simulink model "LKAS_AutoSave_20200908_1055"  (R2018b)
settings: Solver=FixedStepDiscrete  StartTime=0.0  StopTime=10.0  FixedStep=0.01  RelTol=1e-3
InitFcn:
  | tmpVer = ver('MATLAB');
  | tmpVer = str2num(tmpVer.Version);
  | % -------------------------------------------------------------------
  | %  MATLAB file generated by Simulink.saveVars on 21-Nov-2019 10:06:14
  | %  MATLAB version: 7.13.0.564 (R2011b)
  | % -------------------------------------------------------------------
  | 
  | 
  | SInt16 = Simulink.AliasType;
  | SInt16.Description = 'Num';
  | if (tmpVer > 7.11)
  | 	SInt16.DataScope = 'Auto';
  | end
  | SInt16.HeaderFile = 'Rte_Type.h';
  | SInt16.BaseType = 'int16';
  | 
  | SInt32 = Simulink.AliasType;
  | SInt32.Description = 'Num';
  | if (tmpVer > 7.11)
  | 	SInt32.DataScope = 'Auto';
  | end
  | SInt32.HeaderFile = 'Rte_Type.h';
  | SInt32.BaseType = 'int32';
  | 
  | SInt8 = Simulink.AliasType;
  | SInt8.Description = 'Num';
  | if (tmpVer > 7.11)
  | 	SInt8.DataScope = 'Auto';
  | end
  | SInt8.HeaderFile = 'Rte_Type.h';
  | SInt8.BaseType = 'int8';
  | 
  | T_A_m2_1024_1_u32 = Simulink.NumericType;
  | T_A_m2_1024_1_u32.Description = 'm2 (square meters  (m2))';
  | if (tmpVer > 7.11)
  | 	T_A_m2_1024_1_u32.DataScope = 'Auto';
  | end
  | T_A_m2_1024_1_u32.HeaderFile = 'Rte_Type.h';
  | T_A_m2_1024_1_u32.DataTypeMode = 'Fixed-point: slope and bias scaling';
  | T_A_m2_1024_1_u32.SignednessBool = false;
  | T_A_m2_1024_1_u32.WordLength = 32;
  | T_A_m2_1024_1_u32.FixedExponent = -10;
  | T_A_m2_1024_1_u32.SlopeAdjustmentFactor = 1;
  | T_A_m2_1024_1_u32.Bias = 0;
  | T_A_m2_1024_1_u32.DataTypeOverride = 'Inherit';
  | T_A_m2_1024_1_u32.IsAlias = true;
  | 
  | T_A_m2_65536_1_u16 = Simulink.NumericType;
  | T_A_m2_65536_1_u16.Description = 'm2 (square meters  (m2))';
  | if (tmpVer > 7.11)
  | 	T_A_m2_65536_1_u16.DataScope = 'Auto';
  | end
  | T_A_m2_65536_1_u16.HeaderFile = 'Rte_Type.h';
  | T_A_m2_65536_1_u16.DataTypeMode = 'Fixed-point: slope and bias scaling';
  | T_A_m2_65536_1_u16.SignednessBool = false;
  | T_A_m2_65536_1_u16.WordLength = 16;
  | T_A_m2_65536_1_u16.FixedExponent = -16;
  | T_A_m2_65536_1_u16.SlopeAdjustmentFactor = 1;
  | T_A_m2_65536_1_u16.Bias = 0;
  | T_A_m2_65536_1_u16.DataTypeOverride = 'Inherit';
  | ... (+4598 lines)
StopFcn:
  | clear  T_A_m2_1024_1_u32 T_A_m2_65536_1_u16 T_A_m2_Float32 T_A_mm2_10_1_u16 T_A_mm2_4_1_s16 T_A_mm2_Float32 T_Cnt_Num_10_1_u32 T_Cnt_Num_1_1_s16 T_Cnt_Num_1_1_s32 T_Cnt_Num_1_1_s8 T_Cnt_Num_1_1_u16 T_Cnt_Num_1_1_u32 T_Cnt_Num_1_1_u8 T_E_J_1_1_s32 T_E_J_Float32 T_E_kJ_128_1_s32 T_E_kJ_Float32 T_E_kwh_10_1_u16 T_E_kwh_Float32 T_Epl_kwhpkm_100_1_u16 T_Epl_kwhpkm_Float32 T_F_N_1_1_s16 T_F_N_Float32 T_I_A_1000_1_u16 T_I_A_1048576_1_s32 T_I_A_2048_1_s16 T_I_A_32_1_s16 T_I_A_Float32 T_I_mA_1_1_s16 T_I_mA_32768_128_s16 T_I_mA_Float32 T_J_kgpm2_128_1_u16 T_J_kgpm2_Float32 T_K_NA_1000_1_s16 T_K_NA_100_1_s16 T_K_NA_100_1_u16 T_K_NA_1024_1_s16 T_K_NA_1024_1_u16 T_K_NA_128_1_s16 T_K_NA_128_1_u16 T_K_NA_128_1_u8 T_K_NA_16777216_1_u32 T_K_NA_16_1_s16 T_K_NA_16_1_u16 T_K_NA_16_1_u8 T_K_NA_1_16_u16 T_K_NA_1_1_s16 T_K_NA_1_1_u16 T_K_NA_1_1_u8 T_K_NA_32768_1_s16 T_K_NA_32768_1_u16 T_K_NA_32_1_s8 T_K_NA_4096_1_u16 T_K_NA_4194304_1_s32 T_K_NA_4194304_1_u16 T_K_NA_65536_1_s32 T_K_NA_65536_1_u16 T_K_NA_8192_1_s16 T_K_NA_8_1_s16 T_K_NA_Float32 T_M_Nm_16_1_s16 T_M_Nm_1_1_s16 T_M_Nm_32768_1_s16 T_M_Nm_32_1_s16 T_M_Nm_4_1_s16 T_M_Nm_512_1_s16 T_M_Nm_Float32 T_P_W_1_4_s16 T_P_W_1_8_s16 T_P_W_Float32 T_P_kW_128_1_s16 T_P_kW_1_8_s16 T_P_kW_8_1_s32 T_P_kW_Float32 T_Pct_pct_1024_1_s32 T_Pct_pct_1024_1_u32 T_Pct_pct_10_1_s16 T_Pct_pct_10_1_u32 T_Pct_pct_128_100_s8 T_Pct_pct_1_1_s16 T_Pct_pct_1_4_u8 T_Pct_pct_255_100_u16 T_Pct_pct_255_100_u8 T_Pct_pct_256_1_s16 T_Pct_pct_256_1_u16 T_Pct_pct_65535_100_u16 T_Pct_pct_Float32 T_R_ohm_1024_1_s16 T_R_ohm_32_1_s16 T_R_ohm_Float32 T_TK_K_16_1_s16 T_TK_K_Float32 T_T_degC_10_400_1_u16 T_T_degC_16_1_s16 T_T_degC_1_40_1_u8 T_T_degC_2_80_1_u8 T_T_degC_Float32 T_U_V_1000_1_u16 T_U_V_10_1_u8 T_U_V_200_1_u8 T_U_V_32_1_s16 T_U_V_4096_1_s16 T_U_V_512_1_s16 T_U_V_65535_8_u16 T_U_V_8192_1_u16 T_U_V_Float32 T_U_mV_1_1_s16 T_U_mV_256_20_u16 T_U_mV_Float32 T_V_l_256_1_s16 T_V_l_4096_1_s16 T_V_l_64_1_s16 T_V_l_65535_100_u16 T_V_l_Float32 T_V_ml_128_1_s16 T_V_ml_1_1_s16 T_V_ml_32768_1_s16 T_V_ml_Float32 T_V_ul_32_1_u16 T_V_ul_Float32 T_Vpl_clpkm_512_1_u16 T_Vpl_clpkm_Float32 T_a_kphps_16_1_s16 T_a_kphps_Float32 T_a_mps2_128_1_s16 T_a_mps2_Float32 T_c_MJpkg_256_1_s16 T_c_MJpkg_Float32 T_c_kJpgpK_1024_1_s16 T_c_kJpgpK_Float32 T_c_kJpkgpK_128_1_u16 T_c_kJpkgpK_Float32 T_chrg_Ah_1_1_s16 T_chrg_Ah_1_1_u16 T_chrg_Ah_1_1_u8 T_chrg_Ah_256_1_u16 T_chrg_Ah_4194304_1_s32 T_chrg_Ah_512_1_u16 T_chrg_Ah_8_1_u16 T_chrg_Ah_Float32 T_cmp_NA_100_1_s16 T_cmp_NA_128_1_s16 T_cmp_NA_16_1_s16 T_cmp_NA_32768_1_u16 T_cmp_NA_Float32 T_d2n_rpmps2_4_1_s16 T_d2n_rpmps2_Float32 T_dPct_pctps_16_1_s16 T_dPct_pctps_256_1_s16 T_dPct_pctps_Float32 T_dT_degCps_128_1_s16 T_dT_degCps_Float32 T_dV_lph_1_1_s16 T_dV_lph_Float32 T_dV_lpm_128_1_s16 T_dV_lpm_32_1_s16 T_dV_lpm_Float32 T_dV_lps_1024_1_u16 T_dV_lps_4_1_u16 T_dV_lps_Float32 T_dV_mlps_1024_1_s16 T_dV_mlps_Float32 T_d_BitField16 T_dm_gps_128_1_s16 T_dm_gps_128_1_u16 T_dm_gps_256_1_u16 T_dm_gps_Float32 T_dm_mgps_1_1_s16 T_dm_mgps_Float32 T_dn_rpmps_1_1_s16 T_dn_rpmps_2_1_s16 T_dn_rpmps_Float32 T_dp_Paps_1_1_s16 T_dp_Paps_Float32 T_dp_kPaps_1_1_s16 T_dp_kPaps_8_1_s16 T_dp_kPaps_Float32 T_dphi_degps_128_1_s16 T_dphi_degps_8_1_s16 T_dphi_degps_Float32 T_dr_ps_256_1_s16 T_dr_ps_Float32 T_drho_mgplps_1_2_s16 T_drho_mgplps_Float32 T_e_NA_1_1_u8 T_f_Hz_1_1_u16 T_f_Hz_1_1_u32 T_f_Hz_64_1_u16 T_f_Hz_8_1_s16 T_f_Hz_Float32 T_g_BitField32 T_l_km_16_1_s16 T_l_km_1_1_u16 T_l_km_1_1_u32 T_l_km_Float32 T_l_m_1024_1_s16 T_l_m_16_1_s16 T_l_m_1_1_u32 T_l_m_Float32 T_l_mm_16_1_s16 T_l_mm_1_1_u16 T_l_mm_4096_1_s16 T_l_mm_4_1_u8 T_l_mm_64_1_s16 T_l_mm_Float32 T_m_g_1_1_s16 T_m_g_2048_1_s16 T_m_g_32_1_u16 T_m_g_Float32 T_m_kg_1024_1_s16 T_m_kg_1_1_s16 T_m_kg_1_1_u32 T_m_kg_Float32 T_m_mg_128_1_s16 T_m_mg_32_1_s16 T_m_mg_Float32 T_n_rpm_1_1_s16 T_n_rpm_1_25_u8 T_n_rpm_256_50_u16 T_n_rpm_2_25_u8 T_n_rpm_4_1_u16 T_n_rpm_Float32 T_p_MPa_64_1_s16 T_p_MPa_Float32 T_p_Pa_1_1_s16 T_p_Pa_Float32 T_p_kPa_1_10_u16 T_p_kPa_1_1_s16 T_p_kPa_1_1_u8 T_p_kPa_256_1_u16 T_p_kPa_32_1_u16 T_p_kPa_64_1_s16 T_p_kPa_Float32 T_phi_deg_100_1_s16 T_phi_deg_1024_1_s16 T_phi_deg_128_1_s16 T_phi_deg_1_1_u8 T_phi_deg_256_1_s16 T_phi_deg_2_1_s8 T_phi_deg_32_1_s16 T_phi_deg_512_6_s32 T_phi_deg_Float32 T_phi_rad_2048_1_s16 T_phi_rad_Float32 T_r_NA_1024_1_s16 T_r_NA_1024_1_u16 T_r_NA_16384_1_s16 T_r_NA_16_1_s16 T_r_NA_256_1_s8 T_r_NA_256_1_u16 T_r_NA_32768_1_u16 T_r_NA_32_1_u16 T_r_NA_4096_1_s16 T_r_NA_65535_2_u16 T_r_NA_8192_1_u16 T_r_NA_Float32 T_rho_gpl_8192_1_s16 T_rho_gpl_Float32 T_rho_kgpm3_16_1_s16 T_rho_kgpm3_Float32 T_rho_mgpl_1_1_s16 T_rho_mgpl_64_1_s16 T_rho_mgpl_Float32 T_t_hour_1_1_s16 T_t_hour_Float32 T_t_m_1_1_u16 T_t_m_Float32 T_t_ms_1_1_s16 T_t_ms_1_1_u16 T_t_ms_1_1_u32 T_t_ms_4096_1_s16 T_t_ms_64_1_s16 T_t_ms_Float32 T_t_s_1000_1_s16 T_t_s_100_1_s16 T_t_s_10_1_s16 T_t_s_10_1_u16 T_t_s_1_1_s16 T_t_s_1_1_u16 T_t_s_1_1_u32 T_t_s_Float32 T_t_us_10_1_u32 T_t_us_1_1_s16 T_t_us_1_1_u32 T_t_us_1_4_u16 T_t_us_Float32 T_v_kph_1_1_u8 T_v_kph_64_1_s16 T_v_kph_64_1_u16 T_v_kph_Float32 T_v_mps_256_1_s16 T_v_mps_Float32 T_w_radps_32_1_s16 T_w_radps_Float32 T_y_BitField8 T_y_BitFieldDiagProgress T_y_BitFieldDiagStatus T_y_NA_1_1_u8 SInt16 SInt32 SInt8 T_BOOLEAN UInt16 UInt32 UInt8 s16 s32 s8 u16 u32 u8
model workspace (MAT data in the model file):
  MCOS : class17 (value not decoded)
  MCOS : class17 (value not decoded)
  MCOS : class17 (value not decoded)
  MCOS : class17 (value not decoded)
  MCOS : class17 (value not decoded)
  MCOS : class17 (value not decoded)
  MCOS : class17 (value not decoded)
  MCOS : class17 (value not decoded)
  MCOS : class17 (value not decoded)
  MCOS : class17 (value not decoded)
  MCOS : class17 (value not decoded)
  MCOS : class17 (value not decoded)
  MCOS : class17 (value not decoded)
  MCOS : class17 (value not decoded)
  MCOS : class17 (value not decoded)
  MCOS : class17 (value not decoded)
  MCOS : class17 (value not decoded)
  MCOS : class17 (value not decoded)
  MCOS : class17 (value not decoded)
  MCOS : class17 (value not decoded)
  MCOS : class17 (value not decoded)
  MCOS : class17 (value not decoded)
  MCOS : class17 (value not decoded)
  MCOS : class17 (value not decoded)
  MCOS : class17 (value not decoded)
  MCOS : class17 (value not decoded)
  MCOS : class17 (value not decoded)
  MCOS : class17 (value not decoded)
  MCOS : class17 (value not decoded)
  MCOS : class17 (value not decoded)
  MCOS : class17 (value not decoded)
  MCOS : class17 (value not decoded)
  MCOS : class17 (value not decoded)
  MCOS : class17 (value not decoded)
  MCOS : class17 (value not decoded)
  MCOS : class17 (value not decoded)
  MCOS : class17 (value not decoded)
  MCOS : class17 (value not decoded)
  MCOS : class17 (value not decoded)
  MCOS : class17 (value not decoded)
  MCOS : class17 (value not decoded)
  MCOS : class17 (value not decoded)
  MCOS : class17 (value not decoded)
  MCOS : class17 (value not decoded)
  MCOS : class17 (value not decoded)
  MCOS : class17 (value not decoded)
  MCOS : class17 (value not decoded)
  MCOS : class17 (value not decoded)
  MCOS : class17 (value not decoded)
  MCOS : class17 (value not decoded)
  MCOS : class17 (value not decoded)
  MCOS : class17 (value not decoded)
  MCOS : class17 (value not decoded)
  MCOS : class17 (value not decoded)
  MCOS : class17 (value not decoded)
  MCOS : class17 (value not decoded)
  MCOS : class17 (value not decoded)
  MCOS : class17 (value not decoded)
  MCOS : class17 (value not decoded)
  MCOS : class17 (value not decoded)
  MCOS : class17 (value not decoded)
  MCOS : class17 (value not decoded)
  MCOS : class17 (value not decoded)
  MCOS : class17 (value not decoded)
  MCOS : class17 (value not decoded)
  MCOS : class17 (value not decoded)
  MCOS : class17 (value not decoded)
  MCOS : class17 (value not decoded)
  MCOS : class17 (value not decoded)
  MCOS : class17 (value not decoded)
  MCOS : class17 (value not decoded)
  MCOS : class17 (value not decoded)
  MCOS : class17 (value not decoded)
  MCOS : class17 (value not decoded)
  MCOS : class17 (value not decoded)
  MCOS : class17 (value not decoded)
  MCOS : class17 (value not decoded)
  MCOS : class17 (value not decoded)
  MCOS : class17 (value not decoded)
  MCOS : class17 (value not decoded)
  MCOS : class17 (value not decoded)
  MCOS : class17 (value not decoded)
  MCOS : class17 (value not decoded)
  MCOS : class17 (value not decoded)
  MCOS : class17 (value not decoded)
  MCOS : class17 (value not decoded)
  MCOS : class17 (value not decoded)
  MCOS : class17 (value not decoded)
  MCOS : class17 (value not decoded)
undefined symbols (not defined in the file): LKA_CarWidth, LKA_SampleTime, LKA_StrRatio_C, LKA_Veh2CamL_C, LKA_Veh2CamW_C, LKA_WhlBaseL_C, LL_CompSWA_C, LL_CrvtPrvwT_C, LL_DesDvt_C, LL_DvtComp_C, LL_DvtPrvwT_C, LL_DvtSpdDet_vDvtSpdMin_C, LL_HdAgExT_C, LL_HdAgPrvwT_C, LL_LAccMax_C, LL_LAccRMax_C, LL_LDW_EarliestWarnLine_C, LL_LDW_LatestWarnLine_C, LL_LDWS_SUPPRESS_HEADING, LL_LFClb_TFC_DiffCtlBalance, LL_LFClb_TFC_DiffCtrlMaxSWA, LL_LFClb_TFC_DiffCtrlRatio, LL_LFClb_TFC_facmGainLutGain1_C, LL_LFClb_TFC_facmGainLutGain2_C, LL_LFClb_TFC_facmIntegRatio, LL_LFClb_TFC_facmKlat_C, LL_LFClb_TFC_FfCtlRatio_C, LL_LFClb_TFC_phiIntegCtlMaxSWA_C, LL_LFClb_TFC_tiKlatPrvwT_C, LL_LFClb_TFC_vGainLutVehSpdLwr_C, LL_LFClb_TFC_vGainLutVehSpdUpr_C, LL_LKA_EarliestWarnLine_C, LL_LKA_LatestWarnLine_C, LL_LKAExPrcs_ExitC0Dvt, LL_LKAExPrcs_ExitC0Swt, LL_LKAExPrcs_tiExitTime1, LL_LKAExPrcs_tiExitTime2, LL_LKAExPrcs_tiExitTime3, LL_LKAS_OUT_OF_CONTROL_LAT_VEL, LL_LKAS_OUT_OF_CONTROL_TTLC, LL_LKASWASyn_M0, LL_LKASWASyn_M1, LL_LKASWASyn_M2, LL_LKASWASyn_M3K, LL_LKASWASyn_SWAaddMax, LL_LKASWASyn_T2, LL_LKASWASyn_tiTrqSwaRtTime, LL_LKASWASyn_tiTrqSwaTime, LL_LKASWASyn_TrqMax, LL_LKASWASyn_TrqSwaAddSwt, LL_LKASWASyn_TrqSwaRateDiff, LL_LSpdCompT_C, LL_lStpLngth_C, LL_MAX_DELAY_EPSSTAR_TIME, LL_MAX_DRIVER_TORQUE_DISABLE, LL_MAX_DRIVER_TORQUE_ENABLE, LL_MAX_LANE_WIDTH_DISABLE, LL_MAX_LANE_WIDTH_ENABLE, LL_MAX_LAT_ACC_DISABLE, LL_MAX_LAT_ACC_ENABLE ... (+29)
libraries: simulink x134, dspstat3 x3, simulink_extras x1
(part 9 of 19)

== system LKAS_AutoSave_20200908_1055/LKAS/LL/LLOn/LKA/LKA Motion Planning (LKAMP) /Switching Condition (SwtCon) ==
  SwtCon_stLKAActvFlg : Inport
  SwtCon_bsLKAInPInfo : Inport  Port=2
  SwtCon_vVehSpd : Inport  Port=3
  SwtCon_lLaneWidth_C : Inport  Port=4
  SwtCon_lCarWidth_C : Inport  Port=5
  SwtCon_tiHdAgExTime_C : Inport  Port=6
  SwtCon_tiLSpdCompT_C : Inport  Port=7
  Bus Selector1 : BusSelector  OutputSignals=Pr_bsPrInfo.bsPrCrvtInfo.crPrvwCrvt
  Ending Heading Angle Determination (EndHdAgDet) : Subsystem
  If : If  IfExpression=u1==1  ElseIfExpressions=u1==2
  If Action Subsystem : Subsystem  TreatAsAtomicUnit=on
  If Action Subsystem1 : Subsystem  TreatAsAtomicUnit=on
  If Action Subsystem2 : Subsystem  TreatAsAtomicUnit=on
  Merge : Merge  Inputs=3
  Signal Latching : Subsystem  mask(Signal Latching:){LatchTime=1}
      mask prompts: LatchTime "Latch time(-):"
      mask help:
      | If the latch time is not reached, the input signal will just go through the block. If the latch time is reached, the output will be held and do not change again. The latch time is described with the number of the sampling time.
      | ----vcdc.ascl@jlu 19-01-15
  SwtCon_phiHdAgMax : Outport
  wires:
  Bus Selector1/1 -> Ending Heading Angle Determination (EndHdAgDet)/3(EndHdAgDet_crPrvwCrvt)  "<crPrvwCrvt>"
  SwtCon_bsLKAInPInfo/1 -> Bus Selector1/1
  SwtCon_tiLSpdCompT_C/1 -> Ending Heading Angle Determination (EndHdAgDet)/7(EndHdAgDet_tiLSpdCompT_C)
  Signal Latching/1(Out) -> SwtCon_phiHdAgMax/1
  SwtCon_stLKAActvFlg/1 -> Ending Heading Angle Determination (EndHdAgDet)/1(EndHdAgDet_stLKAActvFlg), If/1
  Merge/1 -> Signal Latching/1(In)
  Ending Heading Angle Determination (EndHdAgDet)/1(EndHdAgDet_phiHdAgMax) -> If Action Subsystem/1(In1), If Action Subsystem1/1(In1)
  SwtCon_vVehSpd/1 -> Ending Heading Angle Determination (EndHdAgDet)/2(EndHdAgDet_vVehSpd)
  SwtCon_tiHdAgExTime_C/1 -> Ending Heading Angle Determination (EndHdAgDet)/6(EndHdAgDet_tiHdAgExTime_C)
  SwtCon_lCarWidth_C/1 -> Ending Heading Angle Determination (EndHdAgDet)/5(EndHdAgDet_lCarWidth_C)
  SwtCon_lLaneWidth_C/1 -> Ending Heading Angle Determination (EndHdAgDet)/4(EndHdAgDet_lLaneWidth_C)
  If Action Subsystem2/1(Out1) -> Merge/3
  If/3 -> If Action Subsystem2/Action
  If Action Subsystem1/1(Out1) -> Merge/2
  If/2 -> If Action Subsystem1/Action
  If Action Subsystem/1(Out1) -> Merge/1
  If/1 -> If Action Subsystem/Action

== system LKAS_AutoSave_20200908_1055/LKAS/LL/LLOn/LKA/LKA SWA Limit (LKASWALim)/Rate Limiter Dynamic  ==
  note: Y(k)
  note: U(k)
  up : Inport
  u : Inport  Port=2
  lo : Inport  Port=3
  Add1 : Sum  OutDataTypeStr=uint16
  Constant : Constant  OutDataTypeStr=uint16  SampleTime=-1
  Delay Input2 : UnitDelay  Description=Store in Global RAM  DisableCoverage=on  SampleTime=-1
  Difference Inputs1 : Sum  Description=Add in CPU  DisableCoverage=on  Inputs=+-  OutDataTypeStr=Inherit: Inherit via back propagation
  Difference Inputs2 : Sum  Description=Add in CPU  OutDataTypeStr=Inherit: Inherit via back propagation
  LatchTime_SY : Constant  OutDataTypeStr=uint16  SampleTime=-1
  Memory : Memory  InheritSampleTime=on
  Relational Operator : RelationalOperator  Operator=<=  OutDataTypeStr=boolean  RndMeth=Nearest
  Saturation Dynamic : simulink/Discontinuities/Saturation Dynamic  OutMin=[]  OutMax=[]  OutDataTypeStr=Inherit: Same as second input  OutDataType=fixdt(1, 16)  OutScaling=2^-10  DoSatur=off
  Saturation2 : Saturate  UpperLimit=10000  LowerLimit=0  OutDataTypeStr=uint16
  Switch : Switch  Criteria=u2 > Threshold
  delta fall limit : Product  DisableCoverage=on  Inputs=**  OutDataTypeStr=Inherit: Inherit via back propagation  SaturateOnIntegerOverflow=on
  delta rise limit : Product  DisableCoverage=on  Inputs=**  OutDataTypeStr=Inherit: Inherit via back propagation  SaturateOnIntegerOverflow=on
  sample time : SampleTimeMath  DisableCoverage=on  TsampMathOp=Ts Only  weightValue=1
  Y : Outport
  wires:
  u/1 -> sample time/1, Switch/1, Difference Inputs1/1
  sample time/1 -> delta fall limit/2, delta rise limit/2
  lo/1 -> delta fall limit/1
  up/1 -> delta rise limit/1
  delta rise limit/1 -> Saturation Dynamic/1
  Difference Inputs2/1 -> Y/1, Delay Input2/1
  Saturation Dynamic/1 -> Difference Inputs2/1
  Switch/1 -> Difference Inputs2/2, Difference Inputs1/2  "Y(k-1)"
  Difference Inputs1/1 -> Saturation Dynamic/2  "( U(k) - Y(k-1) )"
  delta fall limit/1 -> Saturation Dynamic/3
  Add1/1 -> Relational Operator/1, Saturation2/1
  Memory/1 -> Add1/2
  Saturation2/1 -> Memory/1
  LatchTime_SY/1 -> Relational Operator/2
  Constant/1 -> Add1/1
  Relational Operator/1 -> Switch/2
  Delay Input2/1 -> Switch/3  "Y(k-1)"

== system LKAS_AutoSave_20200908_1055/LKAS/LL/LLOn/LKA/Lane Following (LF)/Preview Information Calculation (PIC) ==
  PIC_bsLKAInPInfo : Inport
  Add : Sum
  Add1 : Sum
  Add2 : Sum
  Bus Creator1 : BusCreator  Inputs=5
  Bus Selector1 : BusSelector  OutputSignals=Pr_bsPrInfo.bsPrDvtInfo.lPrvwDvtLft,Pr_bsPrInfo.bsPrDvtInfo.lPrvwDvtRgt,Pr_bsPrInfo.bsPrHdAgInfo.phiPrvwHdAgLft,Pr_bsPrInfo.bsPrHdAgInfo.phiPrvwHdAgRgt,Pr_bsPrInfo.bsPrCrvtInfo.crPrvwCrvtLft,Pr_bsPrInfo.bsPrCrvtInfo.crPrvwCrvtRgt,TTLC_bsTTLCInfo.vLft,TTLC_bsTTLCInfo.vRgt
  Gain : Gain  Gain=0.5
  Gain1 : Gain  Gain=0.5
  Gain2 : Gain  Gain=0.5
  PIC_bsPrvwInfo : Outport
  wires:
  Bus Creator1/1 -> PIC_bsPrvwInfo/1
  PIC_bsLKAInPInfo/1 -> Bus Selector1/1
  Bus Selector1/1 -> Add1/1  "<lPrvwDvtLft>"
  Bus Selector1/2 -> Add1/2  "<lPrvwDvtRgt>"
  Add2/1 -> Gain1/1
  Gain1/1 -> Bus Creator1/3  "PIC_crPrvwCrvt"
  Bus Selector1/4 -> Add/2  "<phiPrvwHdAgRgt>"
  Add1/1 -> Gain2/1
  Gain/1 -> Bus Creator1/2  "PIC_phiPrvwHdAg"
  Bus Selector1/6 -> Add2/2  "<crPrvwCrvtRgt>"
  Add/1 -> Gain/1
  Bus Selector1/3 -> Add/1  "<phiPrvwHdAgLft>"
  Bus Selector1/5 -> Add2/1  "<crPrvwCrvtLft>"
  Bus Selector1/7 -> Bus Creator1/4  "<vLft>"
  Bus Selector1/8 -> Bus Creator1/5  "<vRgt>"
  Gain2/1 -> Bus Creator1/1  "PIC_lPrvwDvt"

== system LKAS_AutoSave_20200908_1055/LKAS/LL/LLOn/LKA/Lane Following (LF)/Trajectory Following Control (TFC) ==
  TFC_bsPrvwInfo : Inport
  TFC_bsInInfoSyn : Inport  Port=2
  TFC_bsTFCClb : Inport  Port=3
  TFC_bsConstantClb : Inport  Port=4
  Bus Selector : BusSelector  OutputSignals=PIC_lPrvwDvt,PIC_phiPrvwHdAg,PIC_crPrvwCrvt
  Bus Selector1 : BusSelector  OutputSignals=LL_LFClb_TFC_tiKlatPrvwT_C,LL_LFClb_TFC_facmKlat_C,LL_LFClb_TFC_vGainLutVehSpdLwr_C,LL_LFClb_TFC_vGainLutVehSpdUpr_C,LL_LFClb_TFC_facmGainLutGain1_C,LL_LFClb_TFC_facmGainLutGain2_C,LL_LFClb_TFC_phiIntegCtlMaxSWA_C,LL_LFClb_TFC_facmIntegRatio,LL_LFClb_TFC_DiffCtrlRatio,LL_LFClb_TFC_DiffCtrlMaxSWA,LL_LFClb_TFC_DiffCtlBalance,LL_LFClb_TFC_FfCtlRatio_C
  Bus Selector2 : BusSelector  OutputSignals=LKA_WhlBaseL_C,LKA_StrRatio_C
  Bus Selector3 : BusSelector  OutputSignals=bsLaneInfo.bsL0Info,bsLaneInfo.bsR0Info,bsVehMovInfo.ESC_VehSpd
  Feedback Control (FbCtl) : Subsystem
  Feedforward Control (FfCtl) : Subsystem
  TFC_phiFfSWACmd : Outport
  TFC_phiPropSWACmd : Outport  Port=2
  TFC_phiIntegSWACmd : Outport  Port=3
  TFC_phiDiffSWACmd : Outport  Port=4
  wires:
  Feedback Control (FbCtl)/3(FbCtl_phiFbDiffCtlSWA) -> TFC_phiDiffSWACmd/1
  Bus Selector3/2 -> Feedback Control (FbCtl)/2(FbCtl_bsR0Info)  "<bsR0Info>"
  Bus Selector3/1 -> Feedback Control (FbCtl)/1(FbCtl_bsL0Info)  "<bsL0Info>"
  TFC_bsInInfoSyn/1 -> Bus Selector3/1
  Bus Selector/3 -> Feedforward Control (FfCtl)/3(FfCtl_crPrvwCrvt), Feedback Control (FbCtl)/6(FbCtl_crPrvwCrvt)  "<PIC_crPrvwCrvt>"
  Feedforward Control (FfCtl)/1(FfCtl_phiFfSWA) -> TFC_phiFfSWACmd/1  "phiFfSWA"
  Feedback Control (FbCtl)/1(FbCtl_phiFbPropCtlSWA) -> TFC_phiPropSWACmd/1
  TFC_bsPrvwInfo/1 -> Bus Selector/1  "bsPrvwInfo"
  Bus Selector/1 -> Feedback Control (FbCtl)/4(FbCtl_lPrvwDvt)  "<PIC_lPrvwDvt>"
  Bus Selector/2 -> Feedback Control (FbCtl)/5(FbCtl_phiPrvwHdAg)  "<PIC_phiPrvwHdAg>"
  TFC_bsTFCClb/1 -> Bus Selector1/1
  Bus Selector1/1 -> Feedback Control (FbCtl)/7(FbCtl_tiKlatPrvwT_C)  "<LL_LFClb_TFC_tiKlatPrvwT_C>"
  Bus Selector1/2 -> Feedback Control (FbCtl)/8(FbCtl_facmKlat_C)  "<LL_LFClb_TFC_facmKlat_C>"
  Bus Selector3/3 -> Feedback Control (FbCtl)/3(FbCtl_vVehSpd), Feedforward Control (FfCtl)/2(FfCtl_vVehSpd)  "<ESC_VehSpd>"
  Bus Selector1/3 -> Feedback Control (FbCtl)/9(FbCtl_vVehSpdLimLwr_C)  "<LL_LFClb_TFC_vGainLutVehSpdLwr_C>"
  Bus Selector1/4 -> Feedback Control (FbCtl)/10(FbCtl_vVehSpdLimUpr_C)  "<LL_LFClb_TFC_vGainLutVehSpdUpr_C>"
  Bus Selector1/5 -> Feedback Control (FbCtl)/11(FbCtl_facmGainLimLwr_C)  "<LL_LFClb_TFC_facmGainLutGain1_C>"
  Bus Selector1/6 -> Feedback Control (FbCtl)/12(FbCtl_facmGainLimUpr_C)  "<LL_LFClb_TFC_facmGainLutGain2_C>"
  Bus Selector2/1 -> Feedforward Control (FfCtl)/4(FfCtl_lWhlBase_SY)  "<LKA_WhlBaseL_C>"
  Bus Selector2/2 -> Feedforward Control (FfCtl)/5(FfCtl_rTraRatio_C)  "<LKA_StrRatio_C>"
  TFC_bsConstantClb/1 -> Bus Selector2/1
  Bus Selector1/12 -> Feedforward Control (FfCtl)/1(FfCtl_FfCtlRatio_C)  "<LL_LFClb_TFC_FfCtlRatio_C>"
  Bus Selector1/7 -> Feedback Control (FbCtl)/13(FbCtl_phiIntegCtlMaxSWA_C)  "<LL_LFClb_TFC_phiIntegCtlMaxSWA_C>"
  Bus Selector1/8 -> Feedback Control (FbCtl)/14(FbCtl_facmIntegRatio)  "<LL_LFClb_TFC_facmIntegRatio>"
  Feedback Control (FbCtl)/2(FbCtl_phiFbIntegCtlSWA) -> TFC_phiIntegSWACmd/1
  Bus Selector1/10 -> Feedback Control (FbCtl)/16(FbCtl_DiffCtlMaxSWA)  "<LL_LFClb_TFC_DiffCtrlMaxSWA>"
  Bus Selector1/9 -> Feedback Control (FbCtl)/15(FbCtl_DiffCtlRatioIn)  "<LL_LFClb_TFC_DiffCtrlRatio>"
  Bus Selector1/11 -> Feedback Control (FbCtl)/17(FbCtl_DiffCtlBalance)  "<LL_LFClb_TFC_DiffCtlBalance>"

== system LKAS_AutoSave_20200908_1055/LKAS/LL/LLOn/LKA/Plan To LaneFollowing (PTLF)/InsideJudge ==
  Flg : Inport
  Crvt : Inport  Port=2
  Compare To Constant : simulink/Logic and Bit Operations/Compare To Constant  relop===  const=1  OutDataTypeStr=boolean
  Compare To Constant1 : simulink/Logic and Bit Operations/Compare To Constant  relop===  const=2  OutDataTypeStr=boolean
  Constant : Constant  Value=0.001  OutDataTypeStr=single
  Constant3 : Constant  Value=-0.001  OutDataTypeStr=single
  Logical Operator : Logic  AllPortsSameDT=off  OutDataTypeStr=boolean
  Logical Operator1 : Logic  AllPortsSameDT=off  OutDataTypeStr=boolean
  Logical Operator2 : Logic  Operator=OR  AllPortsSameDT=off  OutDataTypeStr=boolean
  Relational Operator : RelationalOperator  OutDataTypeStr=boolean  RndMeth=Simplest
  Relational Operator1 : RelationalOperator  Operator=<=  OutDataTypeStr=boolean  RndMeth=Simplest
  Out1 : Outport
  wires:
  Compare To Constant/1 -> Logical Operator1/1  "LeftActive"
  Logical Operator1/1 -> Logical Operator2/1
  Logical Operator/1 -> Logical Operator2/2
  Flg/1 -> Compare To Constant1/1, Compare To Constant/1
  Relational Operator/1 -> Logical Operator/2  "RightCrvt"
  Compare To Constant1/1 -> Logical Operator/1  "RightActive"
  Constant/1 -> Relational Operator/2
  Relational Operator1/1 -> Logical Operator1/2  "LeftCrvt"
  Constant3/1 -> Relational Operator1/2
  Logical Operator2/1 -> Out1/1
  Crvt/1 -> Relational Operator1/1, Relational Operator/1

== system LKAS_AutoSave_20200908_1055/LKAS/LL/LLOn/LKA/Plan To LaneFollowing (PTLF)/InsideJudge1 ==
  Flg : Inport
  HdAgLft : Inport  Port=2
  HdAgRgt : Inport  Port=3
  T1 : Inport  Port=4
  Plan : Inport  Port=5
  Time : Inport  Port=6
  If : If  IfExpression=u1 == 1  ElseIfExpressions=u1 == 2
  If Action Subsystem : Subsystem  TreatAsAtomicUnit=on
  If Action Subsystem1 : Subsystem  TreatAsAtomicUnit=on
  If Action Subsystem2 : Subsystem  TreatAsAtomicUnit=on
  Merge : Merge  Inputs=3  InitialOutput=1
  Merge1 : Merge  Inputs=3  InitialOutput=0
  T1_1 : Outport
  Plan_1 : Outport  Port=2
  wires:
  Flg/1 -> If/1
  If/1 -> If Action Subsystem/Action
  If/2 -> If Action Subsystem1/Action
  If/3 -> If Action Subsystem2/Action
  HdAgLft/1 -> If Action Subsystem/3(HdAgLft)
  If Action Subsystem/1(T1_1) -> Merge/1
  If Action Subsystem1/1(T1_1) -> Merge/2
  If Action Subsystem2/1(T1_1) -> Merge/3
  If Action Subsystem/2(Plan_1) -> Merge1/1
  If Action Subsystem1/2(Plan_1) -> Merge1/2
  If Action Subsystem2/2(Plan_1) -> Merge1/3
  T1/1 -> If Action Subsystem/1(T1), If Action Subsystem1/1(T1), If Action Subsystem2/1(T1)
  Plan/1 -> If Action Subsystem/2(Plan), If Action Subsystem1/2(Plan), If Action Subsystem2/2(Plan)
  HdAgRgt/1 -> If Action Subsystem1/3(HdAgRgt)
  Merge/1 -> T1_1/1
  Merge1/1 -> Plan_1/1
  Time/1 -> If Action Subsystem1/4(Time), If Action Subsystem/4(Time)

== system LKAS_AutoSave_20200908_1055/LKAS/LL/LLOn/LKA/Plan To LaneFollowing (PTLF)/LowPass ==
  T : Inport
  u : Inport  Port=2
  dT : Inport  Port=3
  Add : Sum  Inputs=+-
  Add1 : Sum
  Add2 : Sum  OutDataTypeStr=single
  Divide : Product  Inputs=*/
  Divide1 : Product  Inputs=**
  Memory3 : Memory  InheritSampleTime=on
  SWACmdSyn_tiSmplT_C4 : Constant  OutDataTypeStr=single
  Saturation : Saturate  UpperLimit=50  LowerLimit=0
  Switch : Switch  Criteria=u2 > Threshold  Threshold=30
  Unit Delay : UnitDelay  SampleTime=-1
  y : Outport
  wires:
  Switch/1 -> Unit Delay/1, y/1
  Memory3/1 -> Add2/2
  Saturation/1 -> Memory3/1, Switch/2
  Add2/1 -> Saturation/1
  SWACmdSyn_tiSmplT_C4/1 -> Add2/1
  Add1/1 -> Switch/1
  Unit Delay/1 -> Add1/2, Add/2
  Divide1/1 -> Add1/1
  Add/1 -> Divide1/2
  Divide/1 -> Divide1/1
  u/1 -> Add/1, Switch/3
  dT/1 -> Divide/1
  T/1 -> Divide/2

== system LKAS_AutoSave_20200908_1055/LKAS/LL/LLOn/LKA/Plan To LaneFollowing (PTLF)/TickTime (TTime) ==
  Add2 : Sum  OutDataTypeStr=single
  Memory3 : Memory  InheritSampleTime=on
  Saturation : Saturate  UpperLimit=50  LowerLimit=0
  Out1 : Outport
  wires:
  Add2/1 -> Saturation/1
  Memory3/1 -> Add2/2
  Saturation/1 -> Out1/1, Memory3/1
  [LKA_SampleTime] -> Add2/1

== system LKAS_AutoSave_20200908_1055/LKAS/LL/LLOn/LKA/Plan To LaneFollowing (PTLF)/TimeGain ==
  Time : Inport
  T1 : Inport  Port=2
  TFC : Inport  Port=3
  Add1 : Sum
  Add2 : Sum  Inputs=+-
  Add3 : Sum  Inputs=-+
  Constant1 : Constant  Value=0  OutDataTypeStr=single
  Constant4 : Constant  OutDataTypeStr=single
  Divide : Product  Inputs=*/
  Divide8 : Product  Inputs=**
  Saturation4 : Saturate  UpperLimit=1  LowerLimit=0
  Out1 : Outport
  wires:
  Saturation4/1 -> Divide8/2
  Constant1/1 -> Add1/1, Add3/1
  Divide8/1 -> Add1/2
  Add1/1 -> Out1/1
  TFC/1 -> Divide/2
  T1/1 -> Add2/2
  Time/1 -> Add2/1
  Divide/1 -> Saturation4/1
  Add2/1 -> Divide/1
  Constant4/1 -> Add3/2
  Add3/1 -> Divide8/1

== system LKAS_AutoSave_20200908_1055/LKAS/LL/LLOn/LKA Input Processing (LKAInP)/Predicted Deviation Calculation (PrDvt)/Lane Information Selection (LaneInfoSel) ==
  LaneInfoSel_stLKAActvFlg : Inport
  LaneInfoSel_facmLftLane : Inport  Port=2
  LaneInfoSel_facmRgtLane : Inport  Port=3
  If : If  IfExpression=u1==1  ElseIfExpressions=u1==2
  If Action Subsystem1 : Subsystem  TreatAsAtomicUnit=on
  If Action Subsystem2 : Subsystem  TreatAsAtomicUnit=on
  If Action Subsystem3 : Subsystem  TreatAsAtomicUnit=on
  Merge : Merge  Inputs=3
  LaneInfoSel_facmActvLane : Outport
  wires:
  If/3 -> If Action Subsystem3/Action
  If Action Subsystem3/1(Out1) -> Merge/3
  If Action Subsystem1/1(Out1) -> Merge/2
  If/2 -> If Action Subsystem1/Action
  Merge/1 -> LaneInfoSel_facmActvLane/1
  If Action Subsystem2/1(Out1) -> Merge/1
  If/1 -> If Action Subsystem2/Action
  LaneInfoSel_stLKAActvFlg/1 -> If/1
  LaneInfoSel_facmLftLane/1 -> If Action Subsystem3/1(In1), If Action Subsystem2/1(In1)
  LaneInfoSel_facmRgtLane/1 -> If Action Subsystem3/2(In2), If Action Subsystem1/1(In1)

== system LKAS_AutoSave_20200908_1055/LKAS/LL/LLOn/LKA Input Processing (LKAInP)/Predicted Deviation Calculation (PrDvt)/Lane Information Selection (LaneInfoSel)1 ==
  LaneInfoSel_stLKAActvFlg : Inport
  LaneInfoSel_facmLftLane : Inport  Port=2
  LaneInfoSel_facmRgtLane : Inport  Port=3
  If : If  IfExpression=u1==1  ElseIfExpressions=u1==2
  If Action Subsystem1 : Subsystem  TreatAsAtomicUnit=on
  If Action Subsystem2 : Subsystem  TreatAsAtomicUnit=on
  If Action Subsystem3 : Subsystem  TreatAsAtomicUnit=on
  Merge : Merge  Inputs=3
  LaneInfoSel_facmActvLane : Outport
  wires:
  LaneInfoSel_facmRgtLane/1 -> If Action Subsystem1/1(In1), If Action Subsystem3/2(In2)
  LaneInfoSel_facmLftLane/1 -> If Action Subsystem2/1(In1), If Action Subsystem3/1(In1)
  LaneInfoSel_stLKAActvFlg/1 -> If/1
  If/1 -> If Action Subsystem2/Action
  If Action Subsystem2/1(Out1) -> Merge/1
  Merge/1 -> LaneInfoSel_facmActvLane/1
  If/2 -> If Action Subsystem1/Action
  If Action Subsystem1/1(Out1) -> Merge/2
  If Action Subsystem3/1(Out1) -> Merge/3
  If/3 -> If Action Subsystem3/Action

== system LKAS_AutoSave_20200908_1055/LKAS/LL/LLOn/LKA Input Processing (LKAInP)/Predicted Deviation Calculation (PrDvt)/Left Front Conner Deviation Calculation (LFCDvtCalc) ==
  PrdcDvt_bsPrHdAgInfo : Inport
  LFCDvtCalc_lDvt : Inport  Port=2
  LFCDvtCalc_lDvtComp_C : Inport  Port=3
  Add : Sum  Inputs=+-  OutDataTypeStr=single
  Add1 : Sum  OutDataTypeStr=single
  Add5 : Sum  OutDataTypeStr=single
  Bus Selector : BusSelector  OutputSignals=LKA_Veh2CamW_C,LKA_Veh2CamL_C
  Bus Selector2 : BusSelector  OutputSignals=phiHdAgLft
  Cos2 : Trigonometry  Operator=cos
  Divide : Product  Inputs=**
  Divide1 : Product  Inputs=**
  Gain1 : Gain  Gain=-1  OutDataTypeStr=single
  Sin : Trigonometry
  DvtCalc_lLftDvt : Outport
  wires:
  LFCDvtCalc_lDvt/1 -> Add/1
  LFCDvtCalc_lDvtComp_C/1 -> Add/2
  Add/1 -> Add1/1
  Bus Selector/1 -> Add1/2  "<LKA_Veh2CamW_C>"
  [LLClb_bsConstantClb] -> Bus Selector/1
  PrdcDvt_bsPrHdAgInfo/1 -> Bus Selector2/1
  Bus Selector/2 -> Divide1/1  "<LKA_Veh2CamL_C>"
  Bus Selector2/1 -> Sin/1, Cos2/1  "<phiHdAgLft>"
  Gain1/1 -> DvtCalc_lLftDvt/1
  Cos2/1 -> Divide/2
  Sin/1 -> Divide1/2
  Divide/1 -> Add5/1
  Divide1/1 -> Add5/2
  Add1/1 -> Divide/1
  Add5/1 -> Gain1/1

== system LKAS_AutoSave_20200908_1055/LKAS/LL/LLOn/LKA Input Processing (LKAInP)/Predicted Deviation Calculation (PrDvt)/Predicted Deviation Correction (PrdcDvtCor) ==
  PrdcDvtCor_bsPrdcHdAgInfo : Inport
  PrdcDvtCor_lPrvwDstZ : Inport  Port=2
  Bus Selector : BusSelector  OutputSignals=phiPrdcHdAgComp
  Divide2 : Product  Inputs=**  OutDataTypeStr=single
  PrdcDvtCor_lPrdcDvtCor : Outport
  wires:
  Bus Selector/1 -> Divide2/2  "<phiPrdcHdAgComp>"
  PrdcDvtCor_bsPrdcHdAgInfo/1 -> Bus Selector/1
  PrdcDvtCor_lPrvwDstZ/1 -> Divide2/1
  Divide2/1 -> PrdcDvtCor_lPrdcDvtCor/1

== system LKAS_AutoSave_20200908_1055/LKAS/LL/LLOn/LKA Input Processing (LKAInP)/Predicted Deviation Calculation (PrDvt)/Predicted Deviation of Left Lane Line (PrdcDvtLft) ==
  PrdcDvtLft_bsL0Info : Inport
  PrdcDvtLft_lPrvwDstZ : Inport  Port=2
  Add : Sum  Inputs=++++  AccumDataTypeStr=single
  Bus Selector : BusSelector  OutputSignals=L0_C0,L0_C1,L0_C2,L0_C3
  Product : Product  OutDataTypeStr=single  RndMeth=Zero
  Product3 : Product  OutDataTypeStr=single  RndMeth=Zero
  Product4 : Product  OutDataTypeStr=single  RndMeth=Zero
  Z*Z : Product  OutDataTypeStr=single  RndMeth=Zero
  Z*Z*Z : Product  OutDataTypeStr=single  RndMeth=Zero
  PrdcDvtLft_lPrdcDvtLft : Outport
  wires:
  Z*Z/1 -> Z*Z*Z/2, Product3/2
  Z*Z*Z/1 -> Product4/2
  Product4/1 -> Add/4
  Bus Selector/4 -> Product4/1  "<L0_C3>"
  Bus Selector/3 -> Product3/1  "<L0_C2>"
  Product3/1 -> Add/3
  Bus Selector/1 -> Add/1  "<L0_C0>"
  Product/1 -> Add/2
  Bus Selector/2 -> Product/1  "<L0_C1>"
  PrdcDvtLft_lPrvwDstZ/1 -> Z*Z/2, Product/2, Z*Z/1, Z*Z*Z/1
  PrdcDvtLft_bsL0Info/1 -> Bus Selector/1
  Add/1 -> PrdcDvtLft_lPrdcDvtLft/1

== system LKAS_AutoSave_20200908_1055/LKAS/LL/LLOn/LKA Input Processing (LKAInP)/Predicted Deviation Calculation (PrDvt)/Predicted Deviation of Left Line (PrdcDvtLft) ==
  PrdcDvtLft_bsPrdcHdAgInfo : Inport
  PrdcDvtLft_lPrdcDvtCor : Inport  Port=2
  PrdcDvtLft_lPrdcDvtLft : Inport  Port=3
  PrdcDvtLft_lDvtComp_C : Inport  Port=4
  " " : MATLAB Function  TreatAsAtomicUnit=on
  Add : Sum  Inputs=+-  AccumDataTypeStr=single  OutDataTypeStr=single
  Add1 : Sum  AccumDataTypeStr=single  OutDataTypeStr=single
  Add3 : Sum  AccumDataTypeStr=single  OutDataTypeStr=single
  Bus Selector : BusSelector  OutputSignals=phiPrvwTTLCHdAgLft,phiPrdcTTLCHdAg
  Bus Selector1 : BusSelector  OutputSignals=LKA_Veh2CamW_C,LKA_Veh2CamL_C
  Fcn3 : Fcn  Commented=on  Expr=u(2)*cos(u(1))+u(3)*sin(u(1))
  MATLAB Function : MATLAB Function  TreatAsAtomicUnit=on
  PrdcDvtLft_lDvtLft : Outport
  wires:
  Bus Selector1/1 -> " "/2(u2)  "<LKA_Veh2CamW_C>"
  Bus Selector/2 -> " "/1(u1)  "<phiPrdcTTLCHdAg>"
  Bus Selector/1 -> MATLAB Function/2(u2)  "<phiPrvwTTLCHdAgLft>"
  PrdcDvtLft_bsPrdcHdAgInfo/1 -> Bus Selector/1
  Add3/1 -> PrdcDvtLft_lDvtLft/1
  Add1/1 -> Add3/1  "PrvwDvtLft"
  Bus Selector1/2 -> " "/3(u3)  "<LKA_Veh2CamL_C>"
  PrdcDvtLft_lPrdcDvtCor/1 -> Add3/2  "PrdcDvtLft"
  MATLAB Function/1(y) -> Add1/1
  Add/1 -> MATLAB Function/1(u1)
  PrdcDvtLft_lDvtComp_C/1 -> Add/2
  PrdcDvtLft_lPrdcDvtLft/1 -> Add/1
  " "/1(y) -> Add1/2
  [LLClb_bsConstantClb] -> Bus Selector1/1

== system LKAS_AutoSave_20200908_1055/LKAS/LL/LLOn/LKA Input Processing (LKAInP)/Predicted Deviation Calculation (PrDvt)/Predicted Deviation of Right  Line (PrdcDvtRgt) ==
  PrdcDvtLft_bsPrdcHdAgInfo : Inport
  PrdcDvtLft_lPrdcDvtCor : Inport  Port=2
  PrdcDvtLft_lPrdcDvtLft : Inport  Port=3
  PrdcDvtLft_lDvtComp_C : Inport  Port=4
  " " : MATLAB Function  TreatAsAtomicUnit=on
  Add : Sum  Inputs=+-  AccumDataTypeStr=single  OutDataTypeStr=single
  Add2 : Sum  AccumDataTypeStr=single  OutDataTypeStr=single
  Add4 : Sum  Inputs=+-  AccumDataTypeStr=single  OutDataTypeStr=single
  Bus Selector : BusSelector  OutputSignals=phiPrvwTTLCHdAgRgt,phiPrdcTTLCHdAg
  Bus Selector1 : BusSelector  OutputSignals=LKA_Veh2CamW_C,LKA_Veh2CamL_C
  Fcn3 : Fcn  Commented=on  Expr=u(2)*cos(u(1))-u(3)*sin(u(1))
  MATLAB Function : MATLAB Function  TreatAsAtomicUnit=on
  PrdcDvtLft_lDvtRgt : Outport
  wires:
  Bus Selector/2 -> " "/1(u1)  "<phiPrdcTTLCHdAg>"
  Bus Selector/1 -> MATLAB Function/2(u2)  "<phiPrvwTTLCHdAgRgt>"
  PrdcDvtLft_bsPrdcHdAgInfo/1 -> Bus Selector/1
  Add2/1 -> PrdcDvtLft_lDvtRgt/1
  Bus Selector1/2 -> " "/3(u3)  "<LKA_Veh2CamL_C>"
  Bus Selector1/1 -> " "/2(u2)  "<LKA_Veh2CamW_C>"
  MATLAB Function/1(y) -> Add4/1
  Add/1 -> MATLAB Function/1(u1)
  PrdcDvtLft_lDvtComp_C/1 -> Add/2
  PrdcDvtLft_lPrdcDvtLft/1 -> Add/1
  Add4/1 -> Add2/1  "PrvwDvtRgt"
  " "/1(y) -> Add4/2
  PrdcDvtLft_lPrdcDvtCor/1 -> Add2/2  "PrdcDvtRgt"
  [LLClb_bsConstantClb] -> Bus Selector1/1

== system LKAS_AutoSave_20200908_1055/LKAS/LL/LLOn/LKA Input Processing (LKAInP)/Predicted Deviation Calculation (PrDvt)/Predicted Deviation of Right Lane Line (PrdcDvtRgt) ==
  PrdcDvtRgt_lPrvwDstZ : Inport
  PrdcDvtRgt_bsR0Info : Inport  Port=2
  Add : Sum  Inputs=++++  AccumDataTypeStr=single
  Bus Selector : BusSelector  OutputSignals=R0_C0,R0_C1,R0_C2,R0_C3
  Product : Product  OutDataTypeStr=single  RndMeth=Zero
  Product3 : Product  OutDataTypeStr=single  RndMeth=Zero
  Product4 : Product  OutDataTypeStr=single  RndMeth=Zero
  Z*Z : Product  OutDataTypeStr=single  RndMeth=Zero
  Z*Z*Z : Product  OutDataTypeStr=single  RndMeth=Zero
  PrdcDvtRgt_lPrdcDvtRgt : Outport
  wires:
  Z*Z/1 -> Z*Z*Z/2, Product3/2
  Z*Z*Z/1 -> Product4/2
  Product4/1 -> Add/4
  Bus Selector/4 -> Product4/1  "<R0_C3>"
  Bus Selector/3 -> Product3/1  "<R0_C2>"
  Product3/1 -> Add/3
  Bus Selector/1 -> Add/1  "<R0_C0>"
  Add/1 -> PrdcDvtRgt_lPrdcDvtRgt/1
  Product/1 -> Add/2
  Bus Selector/2 -> Product/1  "<R0_C1>"
  PrdcDvtRgt_lPrvwDstZ/1 -> Z*Z/2, Product/2, Z*Z/1, Z*Z*Z/1
  PrdcDvtRgt_bsR0Info/1 -> Bus Selector/1

== system LKAS_AutoSave_20200908_1055/LKAS/LL/LLOn/LKA Input Processing (LKAInP)/Predicted Deviation Calculation (PrDvt)/Right Front Conner Deviation Calculation (RFCDvtCalc) ==
  RFCDvtCalc_lDvtComp_C : Inport
  RFCDvtCalc_lDvt : Inport  Port=2
  PrdcDvt_bsPrHdAgInfo : Inport  Port=3
  Add : Sum  Inputs=+-  OutDataTypeStr=single
  Add1 : Sum  Inputs=+-  OutDataTypeStr=single
  Add5 : Sum  OutDataTypeStr=single
  Bus Selector1 : BusSelector  OutputSignals=LKA_Veh2CamW_C,LKA_Veh2CamL_C
  Bus Selector2 : BusSelector  OutputSignals=phiHdAgRgt
  Cos2 : Trigonometry  Operator=cos
  Divide : Product  Inputs=**
  Divide1 : Product  Inputs=**
  Sin : Trigonometry
  DvtCalc_lRgtDvt : Outport
  wires:
  RFCDvtCalc_lDvt/1 -> Add/1
  RFCDvtCalc_lDvtComp_C/1 -> Add/2
  Add/1 -> Add1/1
  PrdcDvt_bsPrHdAgInfo/1 -> Bus Selector2/1
  Bus Selector1/1 -> Add1/2  "<LKA_Veh2CamW_C>"
  Bus Selector1/2 -> Divide1/1  "<LKA_Veh2CamL_C>"
  [LLClb_bsConstantClb] -> Bus Selector1/1
  Add5/1 -> DvtCalc_lRgtDvt/1
  Sin/1 -> Divide1/2
  Divide1/1 -> Add5/2
  Bus Selector2/1 -> Cos2/1, Sin/1  "<phiHdAgRgt>"
  Cos2/1 -> Divide/2
  Add1/1 -> Divide/1
  Divide/1 -> Add5/1

== system LKAS_AutoSave_20200908_1055/LKAS/LL/LLOn/LKA Input Processing (LKAInP)/Predicted Deviation Calculation (PrDvt)/Z Calculation (ZCalc) ==
  ZCalc_vVehSpd : Inport
  ZCalc_tiDvtPrvwT_C : Inport  Port=2
  Divide : Product  Inputs=**  OutDataTypeStr=single
  kph to mps : Gain  Gain=1/3.6  OutDataTypeStr=single
  ZCalc_lPrvwDstZ : Outport
  wires:
  ZCalc_tiDvtPrvwT_C/1 -> Divide/2
  Divide/1 -> ZCalc_lPrvwDstZ/1
  kph to mps/1 -> Divide/1
  ZCalc_vVehSpd/1 -> kph to mps/1

== system LKAS_AutoSave_20200908_1055/LKAS/LL/LLOn/LKA Input Processing (LKAInP)/Predicted Heading Angle Calculation (PrHdAg)/Heading Angle (HdAg) ==
  HdAg_bsLaneInfo : Inport
  Add : Sum  AccumDataTypeStr=single
  Bus Selector : BusSelector  OutputSignals=bsLaneInfo.bsL0Info.L0_C1,bsLaneInfo.bsR0Info.R0_C1
  Gain : Gain  Gain=0.5
  HdAg_phiHdAg : Outport
  HdAg_phiHdAgLft : Outport  Port=2
  HdAg_phiHdAgRgt : Outport  Port=3
  wires:
  Add/1 -> Gain/1
  HdAg_bsLaneInfo/1 -> Bus Selector/1
  Bus Selector/1 -> HdAg_phiHdAgLft/1, Add/1  "<L0_C1>"
  Bus Selector/2 -> HdAg_phiHdAgRgt/1, Add/2  "<R0_C1>"
  Gain/1 -> HdAg_phiHdAg/1

== system LKAS_AutoSave_20200908_1055/LKAS/LL/LLOn/LKA Input Processing (LKAInP)/Predicted Heading Angle Calculation (PrHdAg)/Lane Information Selection (LaneInfoSel) ==
  LaneInfoSel_stLKAActvFlg : Inport
  LaneInfoSel_facmLftLane : Inport  Port=2
  LaneInfoSel_facmRgtLane : Inport  Port=3
  If : If  IfExpression=u1==1  ElseIfExpressions=u1==2
  If Action Subsystem1 : Subsystem  TreatAsAtomicUnit=on
  If Action Subsystem2 : Subsystem  TreatAsAtomicUnit=on
  If Action Subsystem3 : Subsystem  TreatAsAtomicUnit=on
  Merge : Merge  Inputs=3
  LaneInfoSel_facmActvLane : Outport
  wires:
  If/3 -> If Action Subsystem3/Action
  If Action Subsystem3/1(Out1) -> Merge/3
  If Action Subsystem1/1(Out1) -> Merge/2
  If/2 -> If Action Subsystem1/Action
  Merge/1 -> LaneInfoSel_facmActvLane/1
  If Action Subsystem2/1(Out1) -> Merge/1
  If/1 -> If Action Subsystem2/Action
  LaneInfoSel_stLKAActvFlg/1 -> If/1
  LaneInfoSel_facmLftLane/1 -> If Action Subsystem3/1(In1), If Action Subsystem2/1(In1)
  LaneInfoSel_facmRgtLane/1 -> If Action Subsystem3/2(In2), If Action Subsystem1/1(In1)

== system LKAS_AutoSave_20200908_1055/LKAS/LL/LLOn/LKA Input Processing (LKAInP)/Predicted Heading Angle Calculation (PrHdAg)/Lane Information Selection (LaneInfoSel)1 ==
  LaneInfoSel_stLKAActvFlg : Inport
  LaneInfoSel_facmLftLane : Inport  Port=2
  LaneInfoSel_facmRgtLane : Inport  Port=3
  If : If  IfExpression=u1==1  ElseIfExpressions=u1==2
  If Action Subsystem1 : Subsystem  TreatAsAtomicUnit=on
  If Action Subsystem2 : Subsystem  TreatAsAtomicUnit=on
  If Action Subsystem3 : Subsystem  TreatAsAtomicUnit=on
  Merge : Merge  Inputs=3
  LaneInfoSel_facmActvLane : Outport
  wires:
  LaneInfoSel_facmRgtLane/1 -> If Action Subsystem1/1(In1), If Action Subsystem3/2(In2)
  LaneInfoSel_facmLftLane/1 -> If Action Subsystem2/1(In1), If Action Subsystem3/1(In1)
  LaneInfoSel_stLKAActvFlg/1 -> If/1
  If/1 -> If Action Subsystem2/Action
  If Action Subsystem2/1(Out1) -> Merge/1
  Merge/1 -> LaneInfoSel_facmActvLane/1
  If/2 -> If Action Subsystem1/Action
  If Action Subsystem1/1(Out1) -> Merge/2
  If Action Subsystem3/1(Out1) -> Merge/3
  If/3 -> If Action Subsystem3/Action

== system LKAS_AutoSave_20200908_1055/LKAS/LL/LLOn/LKA Input Processing (LKAInP)/Predicted Heading Angle Calculation (PrHdAg)/Perdicted Heading Angle Compensation (PrdcHdAgComp) ==
  PrdcHdAgComp_vVehSpd : Inport
  PrdcHdAgComp_phiSWA : Inport  Port=2
  PrdcHdAgComp_tiHdAgPrvwT_C : Inport  Port=3
  Bus Selector : BusSelector  OutputSignals=LKA_StrRatio_C
  Divide1 : Product  Inputs=***  OutDataTypeStr=single
  Divide2 : Product  Inputs=*/  OutDataTypeStr=single
  Yaw Rate Stable Gain (YRSG) : Subsystem
  kph To mps : Gain  Gain=pi/180  OutDataTypeStr=single
  PrdcHdAgComp_phiPrdcHdAgComp : Outport
  wires:
  PrdcHdAgComp_vVehSpd/1 -> Yaw Rate Stable Gain (YRSG)/1(YRSG_vVehSpd)
  Yaw Rate Stable Gain (YRSG)/1(YRSG_dphiYRSG) -> Divide1/1
  kph To mps/1 -> Divide1/2
  PrdcHdAgComp_tiHdAgPrvwT_C/1 -> Divide1/3
  Divide1/1 -> Divide2/1
  Divide2/1 -> PrdcHdAgComp_phiPrdcHdAgComp/1
  PrdcHdAgComp_phiSWA/1 -> kph To mps/1
  Bus Selector/1 -> Divide2/2  "<LKA_StrRatio_C>"
  [LLClb_bsConstantClb] -> Bus Selector/1

== system LKAS_AutoSave_20200908_1055/LKAS/LL/LLOn/LKA Input Processing (LKAInP)/Predicted Heading Angle Calculation (PrHdAg)/Perdicted Heading Angle from Right Lane Line (PrdcHdAgRgt) ==
  PrdcHdAgRgt_lPrvwDstZ : Inport
  PrdcHdAgRgt_bsR0Info : Inport  Port=2
  Add : Sum  Inputs=+++  AccumDataTypeStr=single
  Bus Selector : BusSelector  OutputSignals=R0_C1,R0_C2,R0_C3
  Gain : Gain  Gain=2  OutDataTypeStr=single
  Gain1 : Gain  Gain=3  OutDataTypeStr=single
  Product3 : Product  OutDataTypeStr=single  RndMeth=Zero
  Product4 : Product  OutDataTypeStr=single  RndMeth=Zero
  Z*Z : Product  OutDataTypeStr=single  RndMeth=Zero
  PrdcHdAgRgt_phiPrdcHdAgRgt : Outport
  wires:
  Gain1/1 -> Product4/1
  Gain/1 -> Product3/1
  Z*Z/1 -> Product4/2
  Product4/1 -> Add/3
  Bus Selector/3 -> Gain1/1  "<R0_C3>"
  Bus Selector/2 -> Gain/1  "<R0_C2>"
  Product3/1 -> Add/2
  Bus Selector/1 -> Add/1  "<R0_C1>"
  PrdcHdAgRgt_lPrvwDstZ/1 -> Z*Z/2, Product3/2, Z*Z/1
  PrdcHdAgRgt_bsR0Info/1 -> Bus Selector/1
  Add/1 -> PrdcHdAgRgt_phiPrdcHdAgRgt/1

== system LKAS_AutoSave_20200908_1055/LKAS/LL/LLOn/LKA Input Processing (LKAInP)/Predicted Heading Angle Calculation (PrHdAg)/Perdicted Heading Angle from Right Lane Line (PrdcHdAgRgt)1 ==
  PrdcHdAgRgt_lPrvwDstZ : Inport
  PrdcHdAgRgt_bsR0Info : Inport  Port=2
  Add : Sum  Inputs=+++  AccumDataTypeStr=single
  Bus Selector : BusSelector  OutputSignals=R0_C1,R0_C2,R0_C3
  Gain : Gain  Gain=2  OutDataTypeStr=single
  Gain1 : Gain  Gain=3  OutDataTypeStr=single
  Product3 : Product  OutDataTypeStr=single  RndMeth=Zero
  Product4 : Product  OutDataTypeStr=single  RndMeth=Zero
  Z*Z : Product  OutDataTypeStr=single  RndMeth=Zero
  PrdcHdAgRgt_phiPrdcHdAgRgt : Outport
  wires:
  Add/1 -> PrdcHdAgRgt_phiPrdcHdAgRgt/1
  PrdcHdAgRgt_bsR0Info/1 -> Bus Selector/1
  PrdcHdAgRgt_lPrvwDstZ/1 -> Z*Z/1, Product3/2, Z*Z/2
  Bus Selector/1 -> Add/1  "<R0_C1>"
  Product3/1 -> Add/2
  Bus Selector/2 -> Gain/1  "<R0_C2>"
  Bus Selector/3 -> Gain1/1  "<R0_C3>"
  Product4/1 -> Add/3
  Z*Z/1 -> Product4/2
  Gain/1 -> Product3/1
  Gain1/1 -> Product4/1

== system LKAS_AutoSave_20200908_1055/LKAS/LL/LLOn/LKA Input Processing (LKAInP)/Predicted Heading Angle Calculation (PrHdAg)/Predicted Heading Angle from Left Lane Line (PrdcHdAgtLft) ==
  PrdcHdAgtLft_bsL0Info : Inport
  PrdcHdAgtLft_lPrvwDstZ : Inport  Port=2
  Add : Sum  Inputs=+++  AccumDataTypeStr=single
  Bus Selector : BusSelector  OutputSignals=L0_C1,L0_C2,L0_C3
  Gain : Gain  Gain=2  OutDataTypeStr=single
  Gain1 : Gain  Gain=3  OutDataTypeStr=single
  Product3 : Product  OutDataTypeStr=single  RndMeth=Zero
  Product4 : Product  OutDataTypeStr=single  RndMeth=Zero
  Z*Z : Product  OutDataTypeStr=single  RndMeth=Zero
  PrdcHdAgtLft_phiPrdcHdAgLft : Outport
  wires:
  Gain1/1 -> Product4/1
  Gain/1 -> Product3/1
  Z*Z/1 -> Product4/2
  Product4/1 -> Add/3
  Bus Selector/3 -> Gain1/1  "<L0_C3>"
  Bus Selector/2 -> Gain/1  "<L0_C2>"
  Product3/1 -> Add/2
  Bus Selector/1 -> Add/1  "<L0_C1>"
  PrdcHdAgtLft_lPrvwDstZ/1 -> Z*Z/2, Product3/2, Z*Z/1
  PrdcHdAgtLft_bsL0Info/1 -> Bus Selector/1
  Add/1 -> PrdcHdAgtLft_phiPrdcHdAgLft/1

== system LKAS_AutoSave_20200908_1055/LKAS/LL/LLOn/LKA Input Processing (LKAInP)/Predicted Heading Angle Calculation (PrHdAg)/Predicted Heading Angle from Left Lane Line (PrdcHdAgtLft)1 ==
  PrdcHdAgtLft_bsL0Info : Inport
  PrdcHdAgtLft_lPrvwDstZ : Inport  Port=2
  Add : Sum  Inputs=+++  AccumDataTypeStr=single
  Bus Selector : BusSelector  OutputSignals=L0_C1,L0_C2,L0_C3
  Gain : Gain  Gain=2  OutDataTypeStr=single
  Gain1 : Gain  Gain=3  OutDataTypeStr=single
  Product3 : Product  OutDataTypeStr=single  RndMeth=Zero
  Product4 : Product  OutDataTypeStr=single  RndMeth=Zero
  Z*Z : Product  OutDataTypeStr=single  RndMeth=Zero
  PrdcHdAgtLft_phiPrdcHdAgLft : Outport
  wires:
  Add/1 -> PrdcHdAgtLft_phiPrdcHdAgLft/1
  PrdcHdAgtLft_bsL0Info/1 -> Bus Selector/1
  PrdcHdAgtLft_lPrvwDstZ/1 -> Z*Z/1, Product3/2, Z*Z/2
  Bus Selector/1 -> Add/1  "<L0_C1>"
  Product3/1 -> Add/2
  Bus Selector/2 -> Gain/1  "<L0_C2>"
  Bus Selector/3 -> Gain1/1  "<L0_C3>"
  Product4/1 -> Add/3
  Z*Z/1 -> Product4/2
  Gain/1 -> Product3/1
  Gain1/1 -> Product4/1

== system LKAS_AutoSave_20200908_1055/LKAS/LL/LLOn/LKA Input Processing (LKAInP)/Predicted Heading Angle Calculation (PrHdAg)/Z Calculation (ZCalc) ==
  ZCalc_vVehSpd : Inport
  ZCalc_tiHdAgPrvwT_C : Inport  Port=2
  Divide : Product  Inputs=**  OutDataTypeStr=single
  kph to mps : Gain  Gain=1/3.6  OutDataTypeStr=single
  ZCalc_lPrvwDstZ : Outport
  wires:
  kph to mps/1 -> Divide/1
  Divide/1 -> ZCalc_lPrvwDstZ/1
  ZCalc_tiHdAgPrvwT_C/1 -> Divide/2
  ZCalc_vVehSpd/1 -> kph to mps/1

== system LKAS_AutoSave_20200908_1055/LKAS/LL/LLOn/LKA Input Processing (LKAInP)/Predicted Heading Angle Calculation (PrHdAg)/Z Calculation (ZCalc)1 ==
  ZCalc_vVehSpd : Inport
  ZCalc_tiHdAgPrvwT_C : Inport  Port=2
  Divide : Product  Inputs=**  OutDataTypeStr=single
  kph to mps : Gain  Gain=1/3.6  OutDataTypeStr=single
  ZCalc_lPrvwDstZ : Outport
  wires:
  ZCalc_vVehSpd/1 -> kph to mps/1
  ZCalc_tiHdAgPrvwT_C/1 -> Divide/2
  Divide/1 -> ZCalc_lPrvwDstZ/1
  kph to mps/1 -> Divide/1

== system LKAS_AutoSave_20200908_1055/LKAS/LL/LLOn/LKA Input Processing (LKAInP)/Previewed Curvature (PrCrvt)/Curvature Ahead of Left Lane Line (CrvtAhdLft) ==
  CrvtAhdLft_bsL0Info : Inport
  CrvtAhdLft_lPrvwDstZ : Inport  Port=2
  Add : Sum  AccumDataTypeStr=single
  Bus Selector : BusSelector  OutputSignals=L0_C2,L0_C3
  Gain : Gain  Gain=2  OutDataTypeStr=single
  Gain1 : Gain  Gain=6  OutDataTypeStr=single
  Product : Product  OutDataTypeStr=single  RndMeth=Zero
  CrvtAhdLft_crCrvtAhdLft : Outport
  wires:
  Add/1 -> CrvtAhdLft_crCrvtAhdLft/1
  Product/1 -> Add/2
  Gain/1 -> Add/1
  Gain1/1 -> Product/1
  Bus Selector/1 -> Gain/1  "<L0_C2>"
  CrvtAhdLft_lPrvwDstZ/1 -> Product/2
  Bus Selector/2 -> Gain1/1  "<L0_C3>"
  CrvtAhdLft_bsL0Info/1 -> Bus Selector/1

== system LKAS_AutoSave_20200908_1055/LKAS/LL/LLOn/LKA Input Processing (LKAInP)/Previewed Curvature (PrCrvt)/Curvature Ahead of Left Lane Line (CrvtAhdLft)1 ==
  CrvtAhdRgt_lPrvwDstZ : Inport
  CrvtAhdRgt_bsR0Info : Inport  Port=2
  Add : Sum  AccumDataTypeStr=single
  Bus Selector : BusSelector  OutputSignals=R0_C2,R0_C3
  Gain : Gain  Gain=2  OutDataTypeStr=single
  Gain1 : Gain  Gain=6  OutDataTypeStr=single
  Product : Product  OutDataTypeStr=single  RndMeth=Zero
  CrvtAhdRgt_crCrvtAhdRgt : Outport
  wires:
  Add/1 -> CrvtAhdRgt_crCrvtAhdRgt/1
  Product/1 -> Add/2
  Gain/1 -> Add/1
  Gain1/1 -> Product/1
  Bus Selector/1 -> Gain/1  "<R0_C2>"
  CrvtAhdRgt_lPrvwDstZ/1 -> Product/2
  Bus Selector/2 -> Gain1/1  "<R0_C3>"
  CrvtAhdRgt_bsR0Info/1 -> Bus Selector/1

== system LKAS_AutoSave_20200908_1055/LKAS/LL/LLOn/LKA Input Processing (LKAInP)/Previewed Curvature (PrCrvt)/Lane Information Selection (LaneInfoSel) ==
  LaneInfoSel_stLKAActvFlg : Inport
  LaneInfoSel_facmLftLane : Inport  Port=2
  LaneInfoSel_facmRgtLane : Inport  Port=3
  If : If  IfExpression=u1==1  ElseIfExpressions=u1==2
  If Action Subsystem1 : Subsystem  TreatAsAtomicUnit=on
  If Action Subsystem2 : Subsystem  TreatAsAtomicUnit=on
  If Action Subsystem3 : Subsystem  TreatAsAtomicUnit=on
  Merge : Merge  Inputs=3
  LaneInfoSel_facmActvLane : Outport
  wires:
  If/3 -> If Action Subsystem3/Action
  If Action Subsystem3/1(Out1) -> Merge/3
  If Action Subsystem1/1(Out1) -> Merge/2
  If/2 -> If Action Subsystem1/Action
  Merge/1 -> LaneInfoSel_facmActvLane/1
  If Action Subsystem2/1(Out1) -> Merge/1
  If/1 -> If Action Subsystem2/Action
  LaneInfoSel_stLKAActvFlg/1 -> If/1
  LaneInfoSel_facmRgtLane/1 -> If Action Subsystem3/2(In2), If Action Subsystem1/1(In1)
  LaneInfoSel_facmLftLane/1 -> If Action Subsystem3/1(In1), If Action Subsystem2/1(In1)

== system LKAS_AutoSave_20200908_1055/LKAS/LL/LLOn/LKA Input Processing (LKAInP)/Previewed Curvature (PrCrvt)/Z Calculation (ZCalc) ==
  ZCalc_vVehSpd : Inport
  ZCalc_tiCrvtPrvwT_C : Inport  Port=2
  Divide : Product  Inputs=**  OutDataTypeStr=single
  kph to mps : Gain  Gain=1/3.6  OutDataTypeStr=single
  ZCalc_lPrvwDstZ : Outport
  wires:
  Divide/1 -> ZCalc_lPrvwDstZ/1
  kph to mps/1 -> Divide/1
  ZCalc_tiCrvtPrvwT_C/1 -> Divide/2
  ZCalc_vVehSpd/1 -> kph to mps/1
